simulink model "project_work_cancello"  (R2022b)
settings: Solver=FixedStepDiscrete  StartTime=0.0  StopTime=120  FixedStep=0.1  RelTol=1e-3
settings Model: PacingRate=0.010000  Creator=marco  LastModifiedBy=marco
settings OptimizationCC: DefaultParameterBehavior=Inlined  UseDivisionForNetSlopeComputation=on  GainParamInheritBuiltInType=on  UseFloatMulNetSlope=on  InlineInvariantSignals=on  PassReuseOutputArgsAs=Individual arguments  ZeroExternalMemoryAtStartup=off  ZeroInternalMemoryAtStartup=off  NoFixptDivByZeroProtection=on  EfficientFloat2IntCast=on  LifeSpan=1  OptimizeBlockOrder=speed  DifferentSizesBufferReuse=on  EfficientTunableParamExpr=on
settings DebuggingCC: ParameterTunabilityLossMsg=error  SFUnexpectedBacktrackingDiag=warning  SFNoUnconditionalDefaultTransitionDiag=warning
settings HardwareCC: ProdBitPerPointer=32  ProdBitPerSizeT=32  ProdBitPerPtrDiffT=32  ProdLargestAtomicInteger=Long  ProdLargestAtomicFloat=Double  ProdWordSize=32  ProdLongLongMode=on  ProdHWDeviceType=ARM Compatible->ARM Cortex-M
settings SFSimCC: MATLABDynamicMemAlloc=off
settings RTWCC: Description=Embedded Coder  SystemTargetFile=ert.tlc  TemplateMakefile=ert_default_tmf  GenerateReport=on  BuildConfiguration=Debug  LaunchReport=on
settings CodeAppCC: ForceParamTrailComments=on  IgnoreCustomStorageClasses=off  OperatorAnnotations=on  SimulinkDataObjDesc=on  SFDataObjDesc=on  CustomSymbolStrGlobalVar=rt$N$M  CustomSymbolStrType=$N$M  CustomSymbolStrFcn=$N$M$F  CustomSymbolStrMacro=$N$M  InsertBlockDesc=on  EnableCustomComments=on
settings ERTTargetCC: TargetLangStandard=C99 (ISO)  GenerateSampleERTMain=on  IncludeMdlTerminateFcn=off  CombineSignalStateStructs=on  SupportAbsoluteTime=off  PurelyIntegerCode=on  SupportComplex=off  SupportNonInlinedSFcns=on  InlinedParameterPlacement=NonHierarchical  ERTCustomFileTemplate=example_file_process.tlc  ERTFilePackagingFormat=CompactWithDataFile

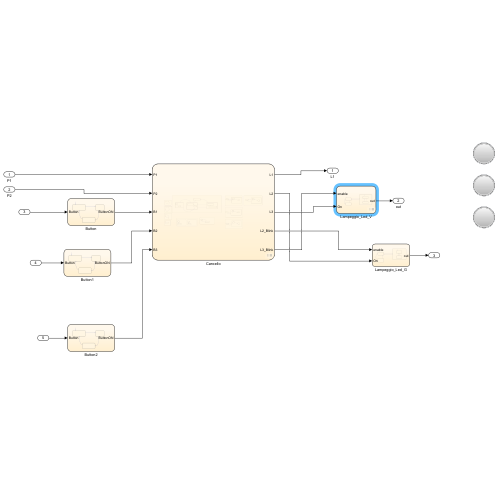
[thumbnail: Simulink's stored preview of the top-level diagram]
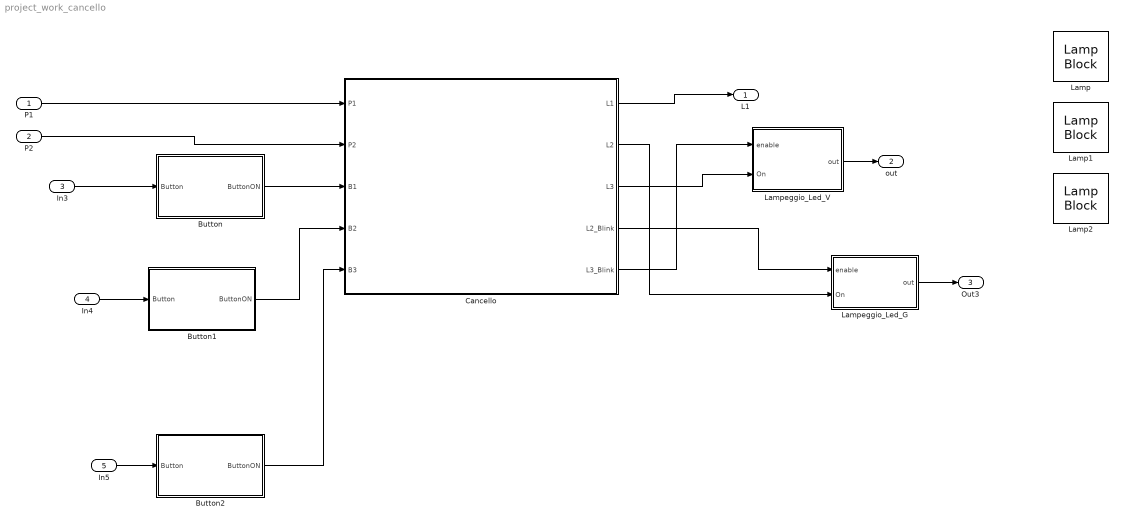
== system project_work_cancello ==
  P1 : Inport
  P2 : Inport  Port=2
  In3 : Inport  Port=3
  In4 : Inport  Port=4
  In5 : Inport  Port=5
  Button : Stateflow chart  TreatAsAtomicUnit=on  SystemSampleTime=0.1
  Button1 : Stateflow chart  TreatAsAtomicUnit=on  SystemSampleTime=0.1
  Button2 : Stateflow chart  TreatAsAtomicUnit=on  SystemSampleTime=0.1
  Cancello : Stateflow chart  TreatAsAtomicUnit=on  SystemSampleTime=0.1
  Lamp : LampBlock  LabelPosition=Hide
  Lamp1 : LampBlock  LabelPosition=Hide
  Lamp2 : LampBlock  LabelPosition=Hide
  Lampeggio_Led_G : Stateflow chart  TreatAsAtomicUnit=on  SystemSampleTime=0.1
  Lampeggio_Led_V : Stateflow chart  TreatAsAtomicUnit=on  SystemSampleTime=0.1
  L1 : Outport
  out : Outport  Port=2
  Out3 : Outport  Port=3
  wires:
  Cancello/5(L3_Blink) -> Lampeggio_Led_V/1(enable)
  Cancello/4(L2_Blink) -> Lampeggio_Led_G/1(enable)
  Cancello/2(L2) -> Lampeggio_Led_G/2(On)
  Cancello/3(L3) -> Lampeggio_Led_V/2(On)
  Button/1(ButtonON) -> Cancello/3(B1)
  Button1/1(ButtonON) -> Cancello/4(B2)
  Button2/1(ButtonON) -> Cancello/5(B3)
  P1/1 -> Cancello/1(P1)
  In3/1 -> Button/1(Button)
  In4/1 -> Button1/1(Button)
  In5/1 -> Button2/1(Button)
  P2/1 -> Cancello/2(P2)
  Cancello/1(L1) -> L1/1
  Lampeggio_Led_V/1(out) -> out/1
  Lampeggio_Led_G/1(out) -> Out3/1

== stateflow chart project_work_cancello/Button ==
  state Wait
    en:ButtonON=Released
  state Pressed
  state LongPressed
    en: ButtonON=Pressed
  (default) -> Wait
  Wait -> Pressed : [Button==Pressed]
  LongPressed -> Wait : [Button==Released]
  Pressed -> LongPressed : [Button==Released]
  data: Button input boolean; ButtonON output boolean; Pressed constant boolean =true; Released constant boolean =false

== stateflow chart project_work_cancello/Button1 ==
  state Wait
    en:ButtonON=Released
  state Pressed
  state LongPressed
    en: ButtonON=Pressed
  (default) -> Wait
  Wait -> Pressed : [Button==Pressed]
  LongPressed -> Wait : [Button==Released]
  Pressed -> LongPressed : [Button==Released]
  data: Button input boolean; ButtonON output boolean; Pressed constant boolean =true; Released constant boolean =false

== stateflow chart project_work_cancello/Cancello ==
  settings: executeAtInitialization=1
  state Cancello [parallel]
    settings: executionOrder=1
    state Check
      en: L1=OFF; L2=OFF; L3=OFF;L2_Blink=OFF;L3_Blink=OFF
    state Error
      state Wait1
      state ERR
        en: L1=ON
        ex: L1=OFF
      (default) -> Wait1
      Wait1 -> ERR : [after(10,sec)]
    state Close
      state Closing
        en:L2_Blink=ON; Start_T_L_C=ON;
        ex:Start_T_L_C=OFF; L2_Blink=OFF;
      state Closed
      (default) -> Closing
      Closing -> Closed : [T_L==ON && P2 == true]
    state Open
      state Opening
        en: Start_T_L_O=ON;L2_Blink=ON;
        ex:L2_Blink=OFF,Start_T_L_O=OFF
      state Opened
        en:L1=ON; L2=ON; L3=ON; Start_T_C=ON;
        du: Reset();
        ex: L1=OFF; L2=OFF; L3=OFF; Start_T_C=OFF;
      (default) -> Opening
      Opening -> Opened : [T_L == ON]
    (default) -> Check
    Check -> Open [order 2] : [B1 == ON && P1 == OFF || P1 == ON && P2 == OFF]
    Close -> Error [order 2] : [T_L==ON&&P2==false]
    Check -> Close [order 1] : [P1 == OFF && P2 == OFF]
    Close -> Open [order 1] : [B1 == ON && P1 == false || in(Close.Closing) && P1==true]
    Error -> Closed : [P2==true]
    Open -> Close : [(B1 == ON || T_C == true) && P1==false]
  state Timer_T_L_O [parallel]
    settings: executionOrder=7
    state Counting
      state Count1
      state End
        en: T_L = ON
      (default) -> Timer_T_L_O.Counting.Count1
      Timer_T_L_O.Counting.Count1 -> Timer_T_L_O.Counting.End [order 1] : [after(Time_T_L,sec)]
      Timer_T_L_O.Counting.Count1 -> Timer_T_L_O.Counting.Count1 [order 2] : [RESET == ON]
    state off
      en: T_L =OFF
    (default) -> Timer_T_L_O.off
    Timer_T_L_O.off -> Timer_T_L_O.Counting : [Start_T_L_O == ON]
    Timer_T_L_O.Counting -> Timer_T_L_O.off : [Start_T_L_O == OFF]
  state Timer_T_L_C [parallel]
    settings: executionOrder=4
    state Counting
      state Count1
      state End
        en: T_L = ON
      (default) -> Timer_T_L_C.Counting.Count1
      Timer_T_L_C.Counting.Count1 -> Timer_T_L_C.Counting.End : [after(Time_T_L,sec)]
    state off
      en: T_L =OFF
    (default) -> Timer_T_L_C.off
    Timer_T_L_C.off -> Timer_T_L_C.Counting : [Start_T_L_C == ON]
    Timer_T_L_C.Counting -> Timer_T_L_C.off : [Start_T_L_C == OFF]
  state Reset [function]
    (default) -> (junction 65)
    (junction 65) -> (junction 68) [order 1] : [P1==true]
    (junction 68) -> (junction 73) : {RESET=true;}
    (junction 65) -> (junction 71) [order 2] : [P1==false]
    (junction 71) -> (junction 73) : {RESET=false;}
  state Update_Time_T_L [function]
    (default) -> (junction 97)
    (junction 97) -> (junction 99) [order 1] : [Time_T_L < 120]
    (junction 99) -> (junction 107) : {Time_T_L=Time_T_L+10}
    (junction 97) -> (junction 103) [order 2] : [Time_T_L >= 120]
    (junction 103) -> (junction 107) : {Time_T_L = 10}
  state Timet_T_C [parallel]
    settings: executionOrder=5
    state Counting
      state Count1
      state End
        en: T_C = ON
      (default) -> Timet_T_C.Counting.Count1
      Timet_T_C.Counting.Count1 -> Timet_T_C.Counting.End [order 1] : [after(Time_T_C,sec)]
      Timet_T_C.Counting.Count1 -> Timet_T_C.Counting.Count1 [order 2] : [RESET == ON]
    state off
      en: T_C =OFF
    (default) -> Timet_T_C.off
    Timet_T_C.off -> Timet_T_C.Counting : [Start_T_C == ON]
    Timet_T_C.Counting -> Timet_T_C.off : [Start_T_C == OFF]
  state Update_Time_T_C [function]
    (default) -> (junction 114)
    (junction 114) -> (junction 116) [order 1] : [Time_T_C < 120]
    (junction 116) -> (junction 120) : {Time_T_C=Time_T_C + 10}
    (junction 114) -> (junction 118) [order 2] : [Time_T_C >= 120]
    (junction 118) -> (junction 120) : {Time_T_C = 10}
  state Obstacle [parallel]
    settings: executionOrder=2
    state Wait
    state OBS
      en: L3_Blink=ON;Start_T_LV=ON
      du: Reset_LV()
      ex:L3_Blink=OFF;Start_T_LV=OFF
    (default) -> Wait
    Wait -> OBS : [(in(Cancello.Close.Closed) || in(Cancello.Open.Opened) || in(Cancello.Check)) && B1==ON &&P1==true]
    OBS -> Wait : [P1==false || T_LV==ON ]
  state Update [parallel]
    settings: executionOrder=3
    state Update_TC [parallel]
      settings: executionOrder=1
      state Update_T_C
      state UP_TC
        en: Update_Time_T_C()
      (default) -> Update_T_C
      UP_TC -> Update_T_C
      Update_T_C -> UP_TC : [(in(Cancello.Close.Closed)||in(Cancello.Check)) && B3 == ON]
    state Update_TL [parallel]
      settings: executionOrder=2
      state Update_T_L
      state UP_TL
        en: Update_Time_T_L()
      (default) -> Update_T_L
      UP_TL -> Update_T_L
      Update_T_L -> UP_TL : [(in(Cancello.Close.Closed) || in(Cancello.Check)) && B2==ON]
  state Timer_LV [parallel]
    settings: executionOrder=6
    state Counting
      state Count1
      state End
        en: T_LV = ON
      (default) -> Timer_LV.Counting.Count1
      Timer_LV.Counting.Count1 -> Timer_LV.Counting.End [order 1] : [after(30,sec)]
      Timer_LV.Counting.Count1 -> Timer_LV.Counting.Count1 [order 2] : [RESET_LV==true]
    state off
      en: T_LV =OFF
    (default) -> Timer_LV.off
    Timer_LV.off -> Timer_LV.Counting : [Start_T_LV == ON]
    Timer_LV.Counting -> Timer_LV.off : [Start_T_LV == OFF]
  state Reset_LV [function]
    (default) -> (junction 81)
    (junction 81) -> (junction 83) [order 1] : [B1==ON]
    (junction 81) -> (junction 89) [order 2] : [B1==OFF]
    (junction 83) -> (junction 87) : {RESET_LV=true}
    (junction 89) -> (junction 87) : {RESET_LV=false}
  data: L1 output boolean; L2 output boolean; L3 output boolean; OFF constant boolean =false; P1 input boolean; P2 input boolean; ON constant boolean =true; B1 input boolean; Time_T_C local int32 =10; Time_T_L local int32 =10; L2_Blink output boolean; L3_Blink output boolean; B2 input boolean; B3 input boolean; RESET local boolean; Start_T_C local boolean; Start_T_L_O local boolean; T_L local boolean; T_C local boolean; T_LV local boolean; RESET_LV local boolean; Start_T_LV local boolean; Start_T_L_C local boolean

== stateflow chart project_work_cancello/Lampeggio_Led_G ==
  state blink
    state blink_on
      en: out = ACTIVE
    state blink_off
      en: out = DISACTIVE
    (default) -> blink_on
    blink_off -> blink_on : after(period, msec)
    blink_on -> blink_off : after(period, msec)
  state off
    en: out = DISACTIVE;
  state on
    en: out=ACTIVE
  (default) -> off
  off -> blink [order 1] : [enable == ACTIVE]
  off -> on [order 2] : [On==ACTIVE]
  blink -> off : [enable == DISACTIVE]
  on -> off : [On==DISACTIVE]
  data: enable input boolean; out output boolean; ACTIVE constant boolean =true; DISACTIVE constant boolean =false; period constant double =2000; On input boolean

== stateflow chart project_work_cancello/Lampeggio_Led_V ==
  state blink
    state blink_on
      en: out = ACTIVE
    state blink_off
      en: out = DISACTIVE
    (default) -> blink_on
    blink_off -> blink_on : after(period, msec)
    blink_on -> blink_off : after(period, msec)
  state off
    en: out = DISACTIVE;
  state on
    en:out = ACTIVE
  (default) -> off
  off -> blink [order 1] : [enable == ACTIVE]
  off -> on [order 2] : [On==ACTIVE]
  blink -> off [order 1] : [enable == DISACTIVE]
  on -> off [order 1] : [On == DISACTIVE]
  blink -> on [order 2] : [enable == DISACTIVE && On == ACTIVE]
  on -> blink [order 2] : [enable == ACTIVE]
  data: enable input boolean; out output boolean; ACTIVE constant boolean =true; DISACTIVE constant boolean =false; period constant double =1000; On input boolean

== stateflow chart project_work_cancello/Button2 ==
  state Wait
    en:ButtonON=Released
  state Pressed
  state LongPressed
    en: ButtonON=Pressed
  (default) -> Wait
  Wait -> Pressed : [Button==Pressed]
  LongPressed -> Wait : [Button==Released]
  Pressed -> LongPressed : [Button==Released]
  data: Button input boolean; ButtonON output boolean; Pressed constant boolean =true; Released constant boolean =false
